simulink model "Nonlinear_Relative_Motion_Equations"  (R2016a)
settings: Solver=ode4  StartTime=0  StopTime=time_end  FixedStep=time_step  MaxStep=0.1  RelTol=1e-12  AbsTol=1e-12
values from neighbouring files (symbols this model uses):
  mu = 398600.4418    [FFNAV_Prop.m]    (also in FFNAV_Troubleshooting.m; Run_NonlinearEquations.m = 398600)
  n = sqrt(mu/a_target^3)    [Run_NonlinearEquations.m]
  rt0 = p_target/(1+e_target*cos(theta0_target))    [Run_NonlinearEquations.m]
  rt_dot0 = sqrt(mu/(a_target*(1-e_target^2)))*e_target*sin(theta0_target)    [Run_NonlinearEquations.m]
  theta0_target = 0    [Run_NonlinearEquations.m]
  theta_dot0 = h_target/rt0^2    [Run_NonlinearEquations.m]
  x0_chaser = .2    (= 0.2)    [Run_NonlinearEquations.m]
  x_dot0_chaser = 0.005    [Run_NonlinearEquations.m]
  y0_chaser = 2*x_dot0_chaser/n    [Run_NonlinearEquations.m]
  y_dot0_chaser = -2*n*x0_chaser    [Run_NonlinearEquations.m]
  z0_chaser = 2*x0_chaser    (= 0.4)    [Run_NonlinearEquations.m]
  z_dot0_chaser = 2*x_dot0_chaser    (= 0.01)    [Run_NonlinearEquations.m]
settings Model: Creator=Cory  LastModifiedBy=Cory
settings DataIOCC: LimitDataPoints=on
settings DebuggingCC: AllowSymbolicDim=off
settings ModelReferenceCC: PropagateSignalLabelsOutOfModel=off
settings GRTTargetCC: GeneratePreprocessorConditionals=Use local settings

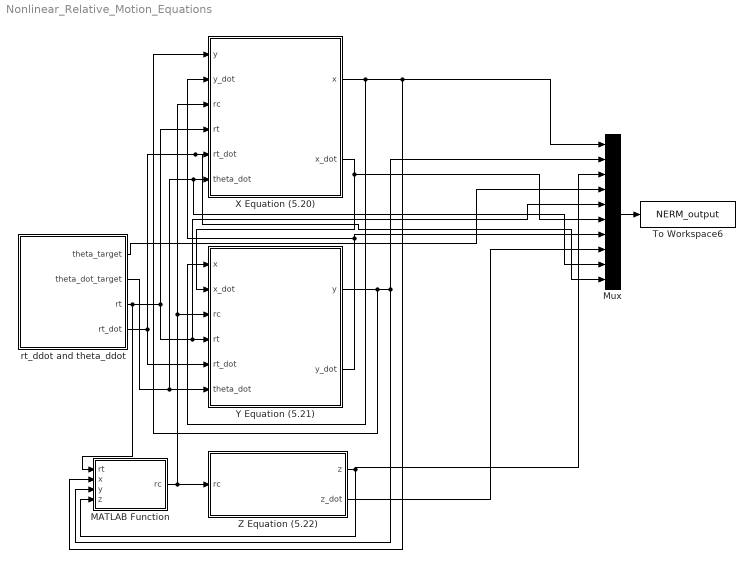
== system Nonlinear_Relative_Motion_Equations ==
  MATLAB Function : MATLAB Function  TreatAsAtomicUnit=on
  Mux : Mux  Inputs=10
  To Workspace6 : ToWorkspace  VariableName=NERM_output  SampleTime=-1
  X Equation (5.20) : Subsystem
  Y Equation (5.21) : Subsystem
  Z Equation (5.22) : Subsystem
  rt_ddot and theta_ddot : Subsystem
  wires:
  X Equation (5.20)/1(x) -> Mux/1, MATLAB Function/2(x), Y Equation (5.21)/1(x)
  rt_ddot and theta_ddot/1(theta_target) -> Mux/4
  Y Equation (5.21)/1(y) -> Mux/2, MATLAB Function/3(y), X Equation (5.20)/1(y)
  Z Equation (5.22)/1(z) -> Mux/3, MATLAB Function/4(z)
  MATLAB Function/1(rc) -> X Equation (5.20)/3(rc), Y Equation (5.21)/3(rc), Z Equation (5.22)/1(rc)
  rt_ddot and theta_ddot/3(rt) -> MATLAB Function/1(rt), Mux/5, Y Equation (5.21)/4(rt), X Equation (5.20)/4(rt)
  rt_ddot and theta_ddot/4(rt_dot) -> Mux/10, X Equation (5.20)/5(rt_dot), Y Equation (5.21)/5(rt_dot)
  rt_ddot and theta_ddot/2(theta_dot_target) -> Mux/9, X Equation (5.20)/6(theta_dot), Y Equation (5.21)/6(theta_dot)
  X Equation (5.20)/2(x_dot) -> Mux/6, Y Equation (5.21)/2(x_dot)
  Y Equation (5.21)/2(y_dot) -> Mux/7, X Equation (5.20)/2(y_dot)
  Mux/1 -> To Workspace6/1
  Z Equation (5.22)/2(z_dot) -> Mux/8

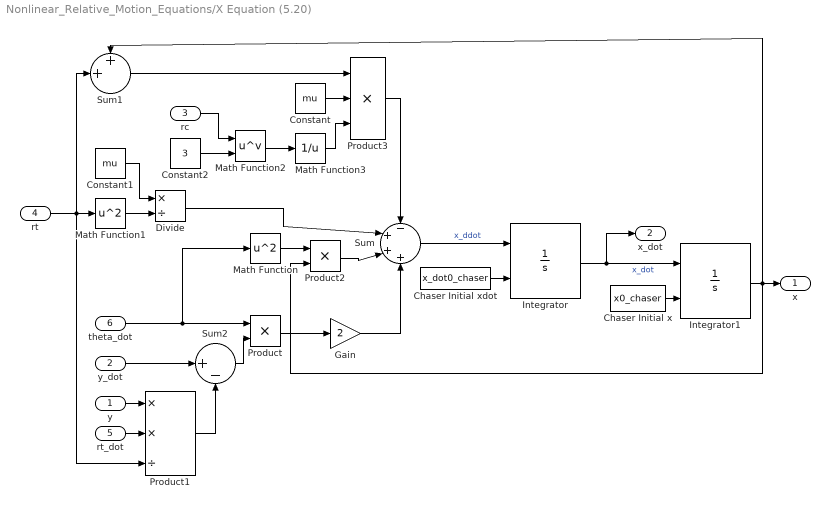
== system Nonlinear_Relative_Motion_Equations/X Equation (5.20) ==
  y : Inport
  y_dot : Inport  Port=2
  rc : Inport  Port=3
  rt : Inport  Port=4
  rt_dot : Inport  Port=5
  theta_dot : Inport  Port=6
  Chaser Initial x : Constant  Value=x0_chaser
  Chaser Initial xdot : Constant  Value=x_dot0_chaser
  Constant : Constant  Value=mu
  Constant1 : Constant  Value=mu
  Constant2 : Constant  Value=3
  Divide : Product  Inputs=*/
  Gain : Gain  Gain=2
  Integrator : Integrator  InitialConditionSource=external
  Integrator1 : Integrator  InitialConditionSource=external
  Math Function : Math  Operator=square  SaturateOnIntegerOverflow=on
  Math Function1 : Math  Operator=square  SaturateOnIntegerOverflow=on
  Math Function2 : Math  Operator=pow  SaturateOnIntegerOverflow=on
  Math Function3 : Math  Operator=reciprocal  SaturateOnIntegerOverflow=on
  Product : Product
  Product1 : Product  Inputs=**/
  Product2 : Product
  Product3 : Product  Inputs=3
  Sum : Sum  Inputs=-+++
  Sum1 : Sum  Inputs=++|
  Sum2 : Sum  Inputs=|+-
  x : Outport
  x_dot : Outport  Port=2
  wires:
  Sum/1 -> Integrator/1  "x_ddot"
  Integrator/1 -> Integrator1/1, x_dot/1  "x_dot"
  Chaser Initial xdot/1 -> Integrator/2
  Constant/1 -> Product3/2
  Integrator1/1 -> Product2/2, Sum1/1, x/1
  rc/1 -> Math Function2/1
  Chaser Initial x/1 -> Integrator1/2
  rt/1 -> Sum1/2, Product1/3, Math Function1/1
  Sum1/1 -> Product3/1
  Constant1/1 -> Divide/1
  Divide/1 -> Sum/2
  Product/1 -> Gain/1
  theta_dot/1 -> Product/1, Math Function/1
  y_dot/1 -> Sum2/1
  y/1 -> Product1/1
  rt_dot/1 -> Product1/2
  Product1/1 -> Sum2/2
  Sum2/1 -> Product/2
  Math Function/1 -> Product2/1
  Product2/1 -> Sum/3
  Gain/1 -> Sum/4
  Math Function1/1 -> Divide/2
  Constant2/1 -> Math Function2/2
  Math Function2/1 -> Math Function3/1
  Math Function3/1 -> Product3/3
  Product3/1 -> Sum/1

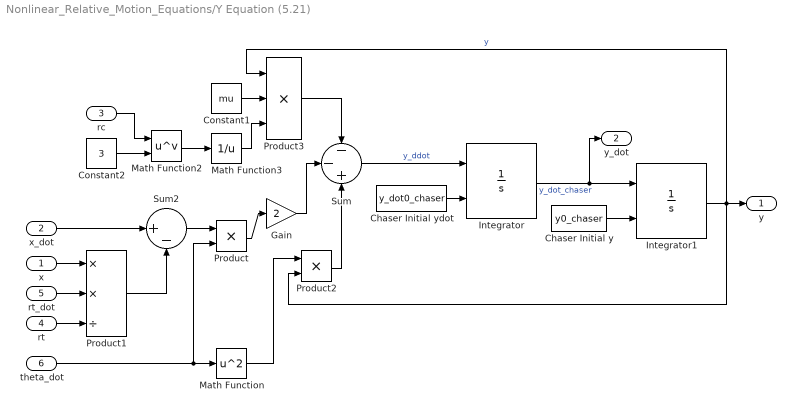
== system Nonlinear_Relative_Motion_Equations/Y Equation (5.21) ==
  x : Inport
  x_dot : Inport  Port=2
  rc : Inport  Port=3
  rt : Inport  Port=4
  rt_dot : Inport  Port=5
  theta_dot : Inport  Port=6
  Chaser Initial y : Constant  Value=y0_chaser
  Chaser Initial ydot : Constant  Value=y_dot0_chaser
  Constant1 : Constant  Value=mu
  Constant2 : Constant  Value=3
  Gain : Gain  Gain=2
  Integrator : Integrator  InitialConditionSource=external
  Integrator1 : Integrator  InitialConditionSource=external
  Math Function : Math  Operator=square  SaturateOnIntegerOverflow=on
  Math Function2 : Math  Operator=pow  SaturateOnIntegerOverflow=on
  Math Function3 : Math  Operator=reciprocal  SaturateOnIntegerOverflow=on
  Product : Product
  Product1 : Product  Inputs=**/
  Product2 : Product
  Product3 : Product  Inputs=3
  Sum : Sum  Inputs=--+
  Sum2 : Sum  Inputs=|+-
  y : Outport
  y_dot : Outport  Port=2
  wires:
  Chaser Initial ydot/1 -> Integrator/2
  Chaser Initial y/1 -> Integrator1/2
  Integrator/1 -> y_dot/1, Integrator1/1  "y_dot_chaser"
  Sum/1 -> Integrator/1  "y_ddot"
  Integrator1/1 -> Product2/2, Product3/1, y/1  "y"
  Product/1 -> Gain/1
  theta_dot/1 -> Product/2, Math Function/1
  Product1/1 -> Sum2/2
  Math Function/1 -> Product2/1
  Gain/1 -> Sum/2
  Product2/1 -> Sum/3
  x_dot/1 -> Sum2/1
  x/1 -> Product1/1
  rt_dot/1 -> Product1/2
  rt/1 -> Product1/3
  Sum2/1 -> Product/1
  Constant1/1 -> Product3/2
  rc/1 -> Math Function2/1
  Constant2/1 -> Math Function2/2
  Math Function2/1 -> Math Function3/1
  Math Function3/1 -> Product3/3
  Product3/1 -> Sum/1

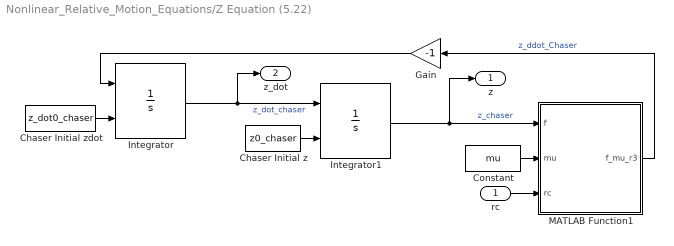
== system Nonlinear_Relative_Motion_Equations/Z Equation (5.22) ==
  rc : Inport
  Chaser Initial z : Constant  Value=z0_chaser
  Chaser Initial zdot : Constant  Value=z_dot0_chaser
  Constant : Constant  Value=mu
  Gain : Gain  Gain=-1
  Integrator : Integrator  InitialConditionSource=external
  Integrator1 : Integrator  InitialConditionSource=external
  MATLAB Function1 : MATLAB Function  TreatAsAtomicUnit=on
  z : Outport
  z_dot : Outport  Port=2
  wires:
  Constant/1 -> MATLAB Function1/2(mu)
  Integrator/1 -> z_dot/1, Integrator1/1  "z_dot_chaser"
  Integrator1/1 -> z/1, MATLAB Function1/1(f)  "z_chaser"
  Gain/1 -> Integrator/1
  MATLAB Function1/1(f_mu_r3) -> Gain/1  "z_ddot_Chaser"
  Chaser Initial zdot/1 -> Integrator/2
  Chaser Initial z/1 -> Integrator1/2
  rc/1 -> MATLAB Function1/3(rc)

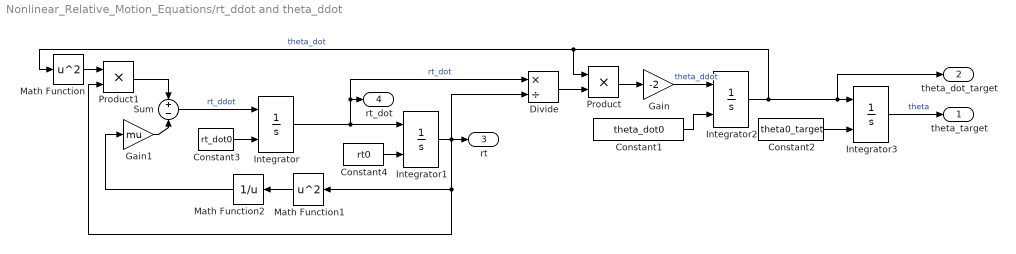
== system Nonlinear_Relative_Motion_Equations/rt_ddot and theta_ddot ==
  Constant1 : Constant  Value=theta_dot0
  Constant2 : Constant  Value=theta0_target
  Constant3 : Constant  Value=rt_dot0
  Constant4 : Constant  Value=rt0
  Divide : Product  Inputs=*/
  Gain : Gain  Gain=-2
  Gain1 : Gain  Gain=mu
  Integrator : Integrator  InitialConditionSource=external
  Integrator1 : Integrator  InitialConditionSource=external
  Integrator2 : Integrator  InitialConditionSource=external  InitialCondition=n
  Integrator3 : Integrator  InitialConditionSource=external
  Math Function : Math  Operator=square  SaturateOnIntegerOverflow=on
  Math Function1 : Math  Operator=square  SaturateOnIntegerOverflow=on
  Math Function2 : Math  Operator=reciprocal  SaturateOnIntegerOverflow=on
  Product : Product
  Product1 : Product
  Sum : Sum  Inputs=+|-
  theta_target : Outport
  theta_dot_target : Outport  Port=2
  rt : Outport  Port=3
  rt_dot : Outport  Port=4
  wires:
  Gain1/1 -> Sum/2
  Math Function2/1 -> Gain1/1
  Math Function1/1 -> Math Function2/1
  Math Function/1 -> Product1/1
  Integrator3/1 -> theta_target/1  "theta"
  Product/1 -> Gain/1
  Sum/1 -> Integrator/1  "rt_ddot"
  Integrator2/1 -> Integrator3/1, theta_dot_target/1, Math Function/1, Product/1  "theta_dot"
  Integrator1/1 -> Product1/2, Math Function1/1, Divide/2, rt/1
  Integrator/1 -> Integrator1/1, Divide/1, rt_dot/1  "rt_dot"
  Divide/1 -> Product/2
  Gain/1 -> Integrator2/1  "theta_ddot"
  Constant1/1 -> Integrator2/2
  Constant2/1 -> Integrator3/2
  Constant3/1 -> Integrator/2
  Constant4/1 -> Integrator1/2
  Product1/1 -> Sum/1

== matlab function Nonlinear_Relative_Motion_Equations/MATLAB Function ==
  data: rt input; x input; y input; z input; rc output
function rc = calc_rc(rt, x, y, z)
%Calculates the radius of the chaser

%Inputs:
%    rt = Target Radius
%    x = Chaser relative x position
%    y = Chaser relative y position
%    z = Chaser relative z position
%Outputs:
%    rc = Chaser Radius

rc = sqrt((rt+x)^2+y^2+z^2);
end

== matlab function Nonlinear_Relative_Motion_Equations/Z Equation (5.22)/MATLAB Function1 ==
  data: f input; f_mu_r3 output; mu input; rc input
function f_mu_r3 = mu_rc3(f, mu, rc)
f_mu_r3 = (mu/rc^3)*f;
end
